simulink model "evaluation_integrator"  (R2014b)
settings: Solver=ode3  SolverMode=SingleTasking  StartTime=0.0  StopTime=Tsim  FixedStep=Ts  RelTol=1e-3
InitFcn:
  | configIntegrator
libraries: simulink x1
settings Model: CovMetricSettings=dwe  CovHtmlReporting=off  covSaveCumulativeToWorkspaceVar=off  CovSaveSingleToWorkspaceVar=off  CovExternalEMLEnable=on  CovSFcnEnable=on  Creator=mnade  LastModifiedBy=nina
settings DataIOCC: LimitDataPoints=off  SaveFormat=StructureWithTime
settings DebuggingCC: SolverPrmCheckMsg=none  FrameProcessingCompatibilityMsg=error  SFUnexpectedBacktrackingDiag=error  SFNoUnconditionalDefaultTransitionDiag=error
settings HardwareCC: ProdBitPerPointer=64  ProdLargestAtomicFloat=Float  ProdIntDivRoundTo=Zero  ProdEndianess=LittleEndian  ProdHWDeviceType=Specified
settings ModelReferenceCC: PropagateSignalLabelsOutOfModel=on
settings GRTTargetCC: TargetLangStandard=C99 (ISO)  GeneratePreprocessorConditionals=Use local settings

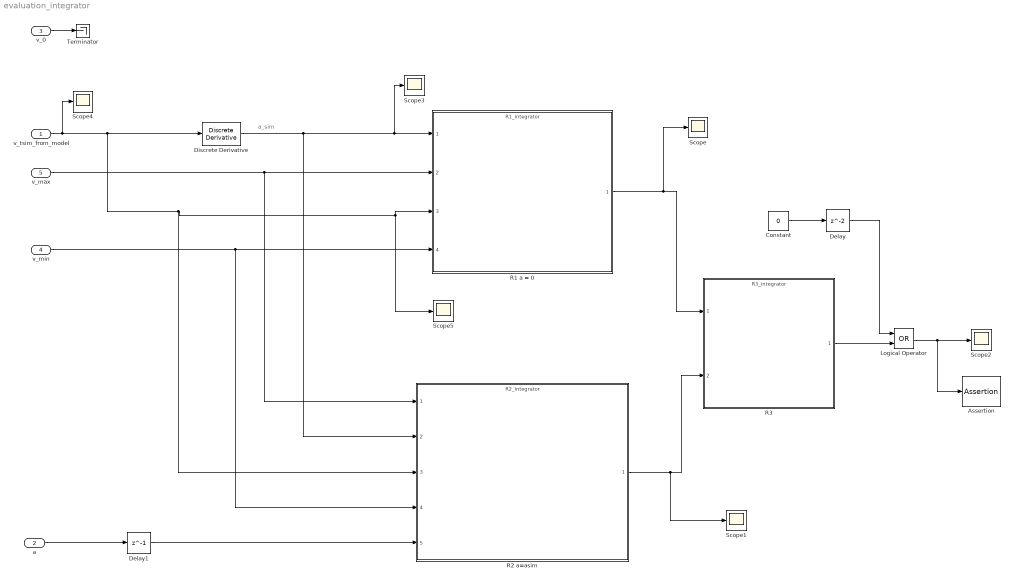
== system evaluation_integrator ==
  note: a_sim
  v_tsim_from_model : Inport
  a : Inport  Port=2
  v_0 : Inport  Port=3
  v_min : Inport  Port=4
  v_max : Inport  Port=5
  Assertion : Assertion  StopWhenAssertionFail=off
  Constant : Constant  Value=0
  Delay : Delay  InitialCondition=1
  Delay1 : Delay  DelayLength=1  InitialCondition=1
  Discrete Derivative : simulink/Discrete/Discrete Derivative  gainval=1.0  ICPrevScaledInput=v_0  OutMin=[]  OutMax=[]  OutDataType=fixdt(1, 16)  OutScaling=2^-10  DoSatur=off
  Logical Operator : Logic  Operator=OR  AllPortsSameDT=off  OutDataTypeStr=boolean
  R1 a = 0 : ModelReference  ModelNameDialog=R1_integrator.slx  SimulationMode=Normal  ModelReferenceVersion=1.29  CopyOfModelName=R1_integrator.slx  DefaultDataLogging=on
  R2 a=asim : ModelReference  ModelNameDialog=R2_integrator.slx  SimulationMode=Normal  ModelReferenceVersion=1.35  CopyOfModelName=R2_integrator.slx  DefaultDataLogging=on
  R3 : ModelReference  ModelNameDialog=R3_integrator.slx  SimulationMode=Normal  ModelReferenceVersion=1.7  CopyOfModelName=R3_integrator.slx  DefaultDataLogging=on
  Scope{,1..5} (6 alike) : Scope
      Scope2 settings: SaveName=ScopeData2
      Scope3 settings: SaveName=ScopeData3
      Scope4 settings: SaveName=ScopeData4
      Scope5 settings: SaveName=ScopeData5
  Terminator : Terminator
  wires:
  R1 a = 0/1 -> Scope/1, R3/1
  v_max/1 -> R2 a=asim/1, R1 a = 0/2
  v_min/1 -> R2 a=asim/4, R1 a = 0/4
  Constant/1 -> Delay/1
  Logical Operator/1 -> Assertion/1, Scope2/1
  R3/1 -> Logical Operator/2
  Delay/1 -> Logical Operator/1
  a/1 -> Delay1/1
  Discrete Derivative/1 -> R2 a=asim/2, Scope3/1, R1 a = 0/1
  v_tsim_from_model/1 -> Scope4/1, Discrete Derivative/1, Scope5/1, R1 a = 0/3, R2 a=asim/3
  v_0/1 -> Terminator/1
  R2 a=asim/1 -> Scope1/1, R3/2
  Delay1/1 -> R2 a=asim/5
